simulink model "desacoplador2"  (R2017a)
settings: Solver=VariableStepAuto  StartTime=0.0  StopTime=10.0  RelTol=1e-3
settings Model: Creator=Lizeth P. Guzman  LastModifiedBy=Lizeth P. Guzman

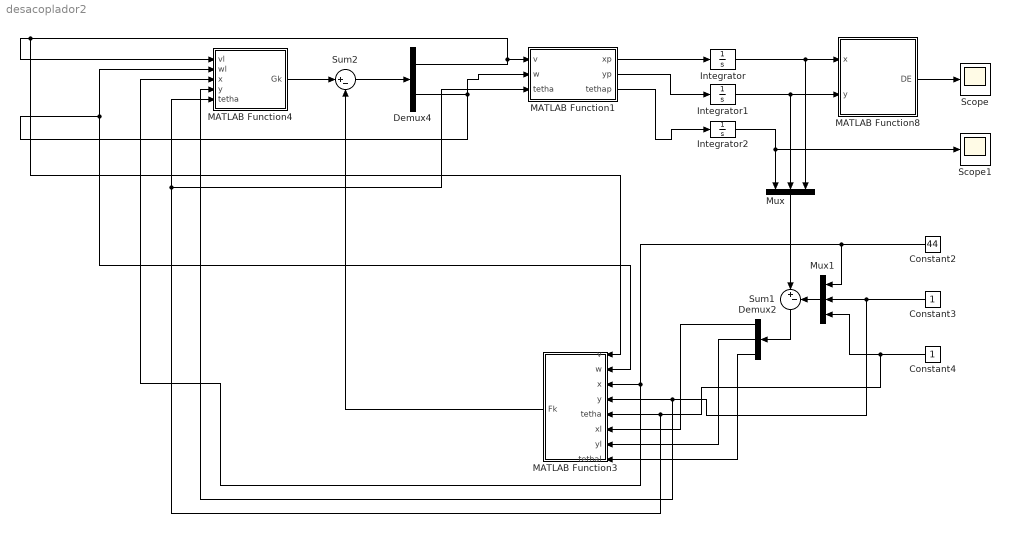
== system desacoplador2 ==
  Constant2 : Constant  Value=44
  Constant3 : Constant
  Constant4 : Constant
  Demux2 : Demux  Outputs=3
  Demux4 : Demux  Outputs=2
  Integrator : Integrator
  Integrator1 : Integrator
  Integrator2 : Integrator
  MATLAB Function1 : MATLAB Function  TreatAsAtomicUnit=on
  MATLAB Function3 : MATLAB Function  TreatAsAtomicUnit=on
  MATLAB Function4 : MATLAB Function  TreatAsAtomicUnit=on
  MATLAB Function8 : MATLAB Function  TreatAsAtomicUnit=on
  Mux : Mux  Inputs=3
  Mux1 : Mux  Inputs=3
  Scope : Scope
  Scope1 : Scope
  Sum1 : Sum  Inputs=|+-
  Sum2 : Sum  Inputs=|+-
  wires:
  MATLAB Function8/1(DE) -> Scope/1
  Sum2/1 -> Demux4/1
  MATLAB Function4/1(Gk) -> Sum2/1
  MATLAB Function3/1(Fk) -> Sum2/2
  MATLAB Function1/1(xp) -> Integrator/1
  MATLAB Function1/2(yp) -> Integrator1/1
  MATLAB Function1/3(tethap) -> Integrator2/1
  Integrator/1 -> Mux/3, MATLAB Function8/1(x)
  Integrator1/1 -> Mux/2, MATLAB Function8/2(y)
  Integrator2/1 -> Mux/1, Scope1/1
  Mux/1 -> Sum1/1
  Constant2/1 -> MATLAB Function4/3(x), MATLAB Function3/3(x), Mux1/1
  Constant3/1 -> MATLAB Function4/4(y), MATLAB Function3/4(y), Mux1/2
  Constant4/1 -> MATLAB Function1/3(tetha), MATLAB Function4/5(tetha), MATLAB Function3/5(tetha), Mux1/3
  Mux1/1 -> Sum1/2
  Sum1/1 -> Demux2/1
  Demux4/1 -> MATLAB Function3/1(v), MATLAB Function4/1(vl), MATLAB Function1/1(v)
  Demux4/2 -> MATLAB Function1/2(w), MATLAB Function3/2(w), MATLAB Function4/2(wl)
  Demux2/1 -> MATLAB Function3/6(xl)
  Demux2/2 -> MATLAB Function3/7(yl)
  Demux2/3 -> MATLAB Function3/8(tethal)

== matlab function desacoplador2/MATLAB Function1 ==
  data: v input; xp output; w input; yp output; tethap output; tetha input
function [xp, yp, tethap] = fcn(v, w, tetha)
%#codegen
d=1;
xp=v*cos(tetha)-d*w*sin(tetha);
yp=v*sin(tetha)+d*w*cos(tetha);
tethap=w;

== matlab function desacoplador2/MATLAB Function3 ==
  data: v input; w input; x input; Fk output; y input; tetha input; xl input; yl input; tethal input
function Fk = fcn(v,w,x, y,tetha, xl, yl, tethal)
%#codegen

d=1;
 
F=[ 0, 0, -((x^2 + y^2)^(1/2)*((x*(v*sin(tetha) + d*w*cos(tetha)))/(x^2 + y^2)^(1/2) - (y*(v*cos(tetha) - d*w*sin(tetha)))/(x^2 + y^2)^(1/2)))/(x*cos(tetha) + y*sin(tetha));
    0, 0,                                                                                                                                                                  0];
k=[xl; yl; tethal];
Fk=F*k;

== matlab function desacoplador2/MATLAB Function4 ==
  data: vl input; wl input; x input; y input; Gk output; tetha input
function  Gk = fcn(vl, wl, x, y, tetha)
%#codegen
d=1;
G =[ (x^2 + y^2)^(1/2)/(x*cos(tetha) + y*sin(tetha)), -(d*(y*cos(tetha) - x*sin(tetha)))/(x*cos(tetha) + y*sin(tetha));
                                                0,                                                                1];
k=[vl;wl];
Gk=G*k;

== matlab function desacoplador2/MATLAB Function8 ==
  data: x input; DE output; y input
function DE = fcn(x, y)
%#codegen

DE=sqrt((x^2)+(y^2));
